simulink model "pend_init_cart"  (R2018b)
settings: Solver=VariableStepAuto  StartTime=0.0  StopTime=T_final  RelTol=1e-3
values from neighbouring files (symbols this model uses):
  adingain = [1 1]    [Parameter_est_brown_rod.mat]    (also in Parameter_est_brown_rod_4.mat; cart_init.mat; fall_blue_rod.mat; fall_blue_rod_2.mat)
  adinoffs = [-0.2676 -0.1653]    [Parameter_est_brown_rod.mat]    (also in Parameter_est_brown_rod_4.mat; cart_init.mat; fall_blue_rod.mat; fall_blue_rod_2.mat)
  angle_bound = [0.287979326579 0 -0.226892802759]    [Parameter_est_brown_rod.mat]    (also in Parameter_est_brown_rod_4.mat; cart_init.mat; fall_blue_rod.mat; fall_blue_rod_2.mat)
  angle_real = [-0.0759 0.0004 0.064]    [Parameter_est_brown_rod.mat]    (also in Parameter_est_brown_rod_4.mat; cart_init.mat; fall_blue_rod.mat; fall_blue_rod_2.mat)
  daoutgain = 0.9    [Parameter_est_brown_rod.mat]    (also in Parameter_est_brown_rod_4.mat; cart_init.mat; fall_blue_rod.mat; fall_blue_rod_2.mat)
  daoutoffs = 0    [Parameter_est_brown_rod.mat]    (also in Parameter_est_brown_rod_4.mat; cart_init.mat; fall_blue_rod.mat; fall_blue_rod_2.mat)
  h = 0.001    [Parameter_Estimation.m]    (also in Parameter_est_brown_rod.mat; Parameter_est_brown_rod_4.mat; cart_init.mat; fall_blue_rod.mat)
  pend = [-0.573 -0.559 -0.487 -0.418 -0.353 -0.29 -0.225 -0.16 -0.094 -0.0247 -0.0037]    [Parameter_est_brown_rod.mat]    (also in Parameter_est_brown_rod_4.mat; cart_init.mat; fall_blue_rod.mat; fall_blue_rod_2.mat)
  u_out = 0.*u_time    [Parameter_Estimation.m]    (also in Parameter_est_brown_rod.mat = [0 5e-07 1.99999999999e-06 4.49999999994e-06 7.99999999966e-; Parameter_est_brown_rod_4.mat = [0 0.00599992500253 0.011998800081 0.0179952756151 0.0239880; cart_init.mat = [0 5e-07 1.99999999999e-06 4.49999999994e-06 7.99999999966e-; fall_blue_rod.mat = [0 0 0 0 0 0 0 0 0 0 0 0 ... (100001 elements, 1x100001)])
  u_time = 0:h:T_final    [Parameter_Estimation.m]    (also in Parameter_est_brown_rod.mat = [0 0.001 0.002 0.003 0.004 0.005 0.006 0.007 0.008 0.009 0.0; Parameter_est_brown_rod_4.mat = [0 0.001 0.002 0.003 0.004 0.005 0.006 0.007 0.008 0.009 0.0; cart_init.mat = [0 0.001 0.002 0.003 0.004 0.005 0.006 0.007 0.008 0.009 0.0; fall_blue_rod.mat = [0 0.001 0.002 0.003 0.004 0.005 0.006 0.007 0.008 0.009 0.0)
undefined symbols (not defined in the file or in its folder): Advantech, PCI
libraries: sldrtlib x2
settings Model: Creator=dvanhanswijk  LastModifiedBy=dvanhanswijk

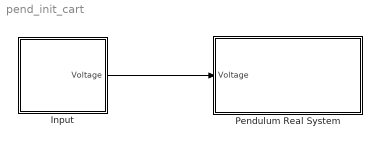
== system pend_init_cart ==
  "Input " : Subsystem
  "Pendulum Real System " : Subsystem
  wires:
  "Input "/1(Voltage) -> "Pendulum Real System "/1(Voltage)

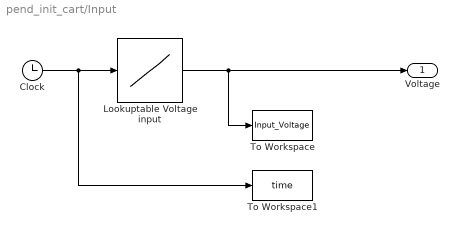
== system pend_init_cart/Input  ==
  Clock : Clock
  Lookuptable Voltage input : Lookup_n-D  NumberOfTableDimensions=1  BreakpointsForDimension1=u_time  Table=u_out  InternalRulePriority=Speed  RndMeth=Simplest  InputSameDT=on
  To Workspace : ToWorkspace  VariableName=Input_Voltage  SaveFormat=Timeseries  SampleTime=-1
  To Workspace1 : ToWorkspace  VariableName=time  SaveFormat=Timeseries  SampleTime=-1
  Voltage : Outport
  wires:
  Lookuptable Voltage input/1 -> To Workspace/1, Voltage/1
  Clock/1 -> Lookuptable Voltage input/1, To Workspace1/1

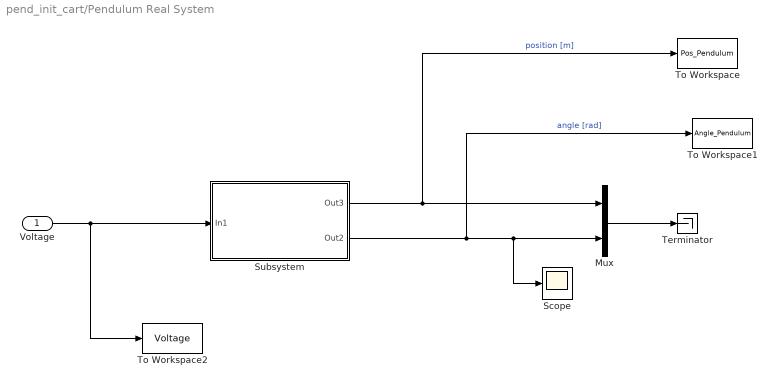
== system pend_init_cart/Pendulum Real System  ==
  Voltage : Inport
  Mux : Mux  Inputs=2
  Scope : Scope
  Subsystem : Subsystem  InitFcn=hwinit  StartFcn=hwinit  mask{h=h}
      mask prompts: h "Sample time"
      mask init:
      | hwinit
      mask Display: disp('Pendulum');
  Terminator : Terminator
  To Workspace : ToWorkspace  VariableName=Pos_Pendulum  SaveFormat=Timeseries  SampleTime=-1
  To Workspace1 : ToWorkspace  VariableName=Angle_Pendulum  SaveFormat=Timeseries  SampleTime=-1
  To Workspace2 : ToWorkspace  VariableName=Voltage  SaveFormat=Timeseries  SampleTime=-1
  wires:
  Mux/1 -> Terminator/1
  Subsystem/2(Out2) -> To Workspace1/1, Scope/1, Mux/2  "angle [rad]"
  Subsystem/1(Out3) -> To Workspace/1, Mux/1  "position [m]"
  Voltage/1 -> Subsystem/1(In1), To Workspace2/1

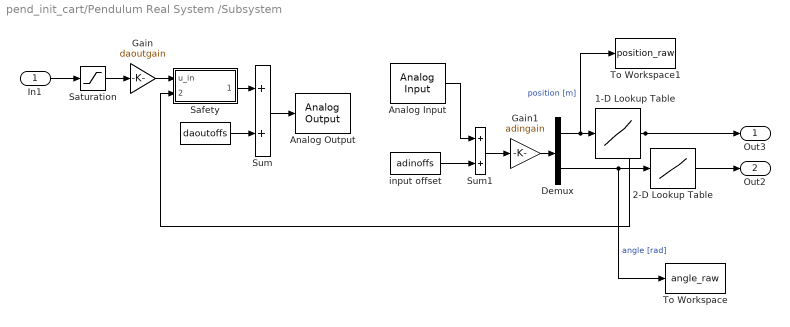
== system pend_init_cart/Pendulum Real System /Subsystem ==
  In1 : Inport
  " " : Constant  Value=daoutoffs
  1-D Lookup Table : Lookup_n-D  NumberOfTableDimensions=1  BreakpointsForDimension1=pend  Table=real  InternalRulePriority=Speed  RndMeth=Simplest  InputSameDT=on
  2-D Lookup Table : Lookup_n-D  NumberOfTableDimensions=1  BreakpointsForDimension1=angle_real  BreakpointsForDimension2=[1:3]  Table=angle_bound  InternalRulePriority=Speed  RndMeth=Simplest  InputSameDT=on
  Analog Input : sldrtlib/Analog Input  SampleTime=h  MaxMissedTicks=ticklost  ShowMissedTicks=off  YieldWhenWaiting=on  DrvName=Advantech/PCI-1711  DrvAddress=4294967295  DrvOptions=zeros(1,0)  Channels=adinchannels  RangeMode=2  VoltRange=1  DataType=1
      settings: AttributesFormatString=Advantech\nPCI-1711 [auto]  SourceProductName=Simulink Desktop Real-Time
  Analog Output : sldrtlib/Analog Output  SampleTime=h  MaxMissedTicks=ticklost  ShowMissedTicks=off  YieldWhenWaiting=off  DrvName=Advantech/PCI-1711  DrvAddress=4294967295  DrvOptions=zeros(1,0)  Channels=daoutchannels  RangeMode=2  VoltRange=2  InitialValue=0  FinalValue=0
      settings: AttributesFormatString=Advantech\nPCI-1711 [auto]  SourceProductName=Simulink Desktop Real-Time
  Demux : Demux  Outputs=2
  Gain : Gain  Gain=daoutgain  SaturateOnIntegerOverflow=on  OutDataTypeStr=Inherit: Same as input  ParamDataTypeStr=Inherit: Same as input
  Gain1 : Gain  Gain=adingain  SaturateOnIntegerOverflow=on  OutDataTypeStr=Inherit: Same as input  ParamDataTypeStr=Inherit: Same as input
  Safety : Subsystem
      mask help: The output of the block is restricted to prevent damage to the system. If the cart reaches some safety margins (left: -0.26 and right: 0.26), the output of the block is nullifed. Then the control has to be restarted.
      mask Display: disp('Safety \n margins')
  Saturation : Saturate  UpperLimit=1  LowerLimit=-1
  Sum : Sum  SaturateOnIntegerOverflow=on  OutDataTypeStr=Inherit: Same as first input
  Sum1 : Sum  SaturateOnIntegerOverflow=on  InputSameDT=on  OutDataTypeStr=Inherit: Same as first input
  To Workspace : ToWorkspace  VariableName=angle_raw  SaveFormat=Timeseries  SampleTime=-1
  To Workspace1 : ToWorkspace  VariableName=position_raw  SaveFormat=Timeseries  SampleTime=-1
  input offset : Constant  Value=adinoffs
  Out3 : Outport
  Out2 : Outport  Port=2
  wires:
  2-D Lookup Table/1 -> Out2/1
  1-D Lookup Table/1 -> Out3/1, Safety/2(Position)
  Demux/1 -> 1-D Lookup Table/1, To Workspace1/1  "position [m]"
  Gain/1 -> Safety/1(u_in)
  Safety/1(u_out) -> Sum/1
  Demux/2 -> To Workspace/1, 2-D Lookup Table/1  "angle [rad]"
  In1/1 -> Saturation/1
  " "/1 -> Sum/2
  Sum/1 -> Analog Output/1
  Saturation/1 -> Gain/1
  Gain1/1 -> Demux/1
  Analog Input/1 -> Sum1/1
  input offset/1 -> Sum1/2
  Sum1/1 -> Gain1/1

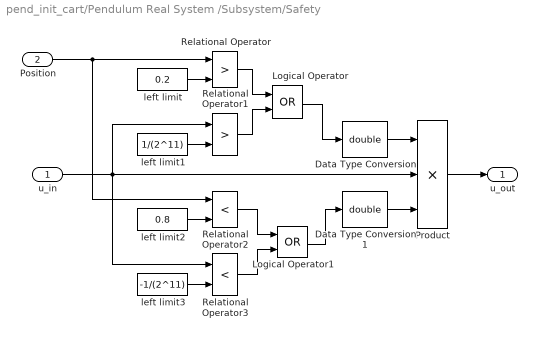
== system pend_init_cart/Pendulum Real System /Subsystem/Safety ==
  u_in : Inport
  Position : Inport  Port=2
  Data Type Conversion : DataTypeConversion  OutDataTypeStr=double
  Data Type Conversion1 : DataTypeConversion  OutDataTypeStr=double
  Logical Operator : Logic  Operator=OR  OutDataTypeStr=boolean
  Logical Operator1 : Logic  Operator=OR  OutDataTypeStr=boolean
  Product : Product  Inputs=3  SaturateOnIntegerOverflow=on  InputSameDT=on  OutDataTypeStr=Inherit: Same as first input
  Relational Operator : RelationalOperator  Operator=>  OutDataTypeStr=boolean  RndMeth=Nearest  InputSameDT=on
  Relational Operator1 : RelationalOperator  Operator=>  OutDataTypeStr=boolean  RndMeth=Nearest  InputSameDT=on
  Relational Operator2 : RelationalOperator  Operator=<  OutDataTypeStr=boolean  RndMeth=Nearest  InputSameDT=on
  Relational Operator3 : RelationalOperator  Operator=<  OutDataTypeStr=boolean  RndMeth=Nearest  InputSameDT=on
  left limit : Constant  Value=0.2
  left limit1 : Constant  Value=1/(2^11)
  left limit2 : Constant  Value=0.8
  left limit3 : Constant  Value=-1/(2^11)
  u_out : Outport
  wires:
  Data Type Conversion1/1 -> Product/3
  Data Type Conversion/1 -> Product/1
  Product/1 -> u_out/1
  Relational Operator3/1 -> Logical Operator1/2
  left limit3/1 -> Relational Operator3/2
  Relational Operator2/1 -> Logical Operator1/1
  left limit2/1 -> Relational Operator2/2
  Position/1 -> Relational Operator2/1, Relational Operator/1
  Relational Operator1/1 -> Logical Operator/2
  Relational Operator/1 -> Logical Operator/1
  left limit/1 -> Relational Operator/2
  Logical Operator/1 -> Data Type Conversion/1
  Logical Operator1/1 -> Data Type Conversion1/1
  u_in/1 -> Product/2, Relational Operator3/1, Relational Operator1/1
  left limit1/1 -> Relational Operator1/2
